simulink model "sbvf_model_2019b_local"  (R2019b)
settings: Solver=VariableStepAuto  StartTime=0.0  StopTime=Tsim  RelTol=1e-3
undefined symbols (not defined in the file): A0, Ad, B, C, c, D, F_local, Gdiag, k, K, L_leader, std_dev, x0, x0_leader
libraries: dspindex x54
settings Model: Creator=andre  LastModifiedBy=frare
settings DebuggingCC: UnconnectedInputMsg=none  UnconnectedOutputMsg=none  UnconnectedLineMsg=none
settings ModelReferenceCC: EnableRefExpFcnMdlSchedulingChecks=off
settings RTWCC: Description=Generic Real-Time Target

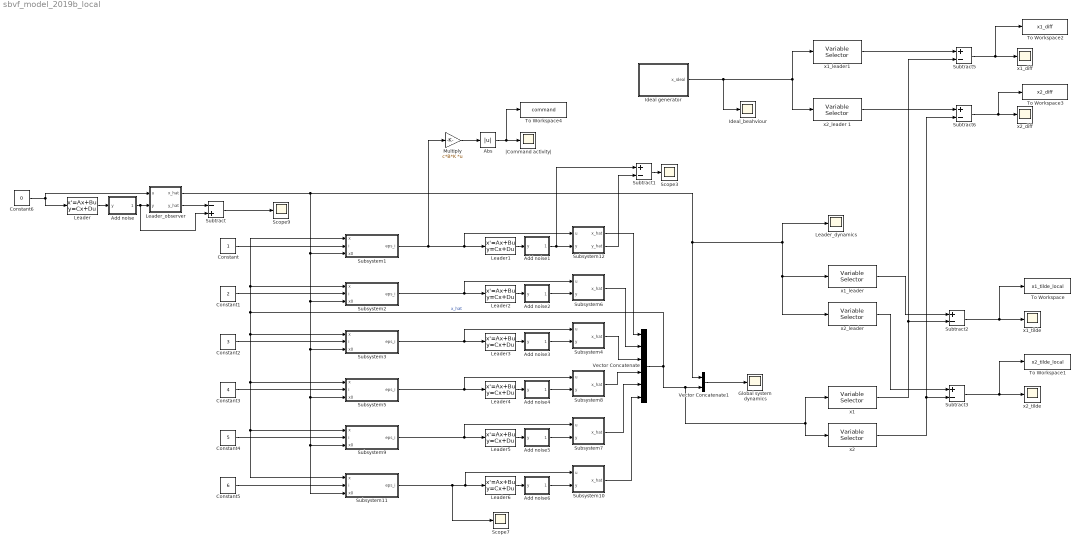
== system sbvf_model_2019b_local ==
  Abs : Abs
  Add noise : Subsystem
  Add noise1 : Subsystem
  Add noise2 : Subsystem
  Add noise3 : Subsystem
  Add noise4 : Subsystem
  Add noise5 : Subsystem
  Add noise6 : Subsystem
  Constant : Constant
  Constant1 : Constant  Value=2
  Constant2 : Constant  Value=3
  Constant3 : Constant  Value=4
  Constant4 : Constant  Value=5
  Constant5 : Constant  Value=6
  Constant6 : Constant  Value=0
  Global system dynamics : Scope
  "Ideal generator " : Subsystem
  "Ideal_beahviour " : Scope
  Leader : StateSpace  A=A0  B=B  C=C  D=0  InitialCondition=x0_leader
  Leader1 : StateSpace  A=A0  B=c*B*K  C=C  D=D  InitialCondition=x0(:,1)
  Leader2 : StateSpace  A=A0  B=c*B*K  C=C  D=D  InitialCondition=x0(:,2)
  Leader3 : StateSpace  A=A0  B=c*B*K  C=C  D=D  InitialCondition=x0(:,3)
  Leader4 : StateSpace  A=A0  B=c*B*K  C=C  D=D  InitialCondition=x0(:,4)
  Leader5 : StateSpace  A=A0  B=c*B*K  C=C  D=D  InitialCondition=x0(:,5)
  Leader6 : StateSpace  A=A0  B=c*B*K  C=C  D=D  InitialCondition=x0(:,6)
  "Leader_dynamics " : Scope
  Leader_observer : Subsystem
  Multiply : Gain  Gain=c*B*K  Multiplication=Matrix(K*u)
  Scope3 : Scope
  Scope7 : Scope
  Scope9 : Scope
  Subsystem1 : Subsystem
  Subsystem10 : Subsystem
  Subsystem11 : Subsystem
  Subsystem12 : Subsystem
  Subsystem2 : Subsystem
  Subsystem3 : Subsystem
  Subsystem4 : Subsystem
  Subsystem5 : Subsystem
  Subsystem6 : Subsystem
  Subsystem7 : Subsystem
  Subsystem8 : Subsystem
  Subsystem9 : Subsystem
  Subtract : Sum  Inputs=-+
  Subtract{1..3,5..6} (5 alike) : Sum  Inputs=+-
  To Workspace : ToWorkspace  VariableName=x1_tilde_local  SaveFormat=Timeseries  SampleTime=-1
  To Workspace1 : ToWorkspace  VariableName=x2_tilde_local  SaveFormat=Timeseries  SampleTime=-1
  To Workspace2 : ToWorkspace  VariableName=x1_diff  SaveFormat=Timeseries  SampleTime=-1
  To Workspace3 : ToWorkspace  VariableName=x2_diff  SaveFormat=Timeseries  SampleTime=-1
  To Workspace4 : ToWorkspace  VariableName=command  SaveFormat=Timeseries  SampleTime=-1
  Vector Concatenate : Concatenate  NumInputs=6  Mode=Multidimensional array  ConcatenateDimension=2
  Vector Concatenate1 : Concatenate  Mode=Multidimensional array  ConcatenateDimension=2
  "x1 " : dspindex/Variable Selector  NumInputs=1  rowsOrCols=Rows  IdxMode=Fixed  Elements=1  ZerOneIdxMode=One-based  errmode=Clip Index  FillMode=on  FillValues=0
  "x1_diff " : Scope
  x1_leader : dspindex/Variable Selector  NumInputs=1  rowsOrCols=Rows  IdxMode=Fixed  Elements=1  ZerOneIdxMode=One-based  errmode=Clip Index  FillMode=on  FillValues=0
  x1_leader1 : dspindex/Variable Selector  NumInputs=1  rowsOrCols=Rows  IdxMode=Fixed  Elements=1  ZerOneIdxMode=One-based  errmode=Clip Index  FillMode=on  FillValues=0
  x1_tilde : Scope
  x2 : dspindex/Variable Selector  NumInputs=1  rowsOrCols=Rows  IdxMode=Fixed  Elements=2  ZerOneIdxMode=One-based  errmode=Clip Index  FillMode=on  FillValues=0
  x2_diff : Scope
  "x2_leader " : dspindex/Variable Selector  NumInputs=1  rowsOrCols=Rows  IdxMode=Fixed  Elements=2  ZerOneIdxMode=One-based  errmode=Clip Index  FillMode=on  FillValues=0
  x2_leader 1 : dspindex/Variable Selector  NumInputs=1  rowsOrCols=Rows  IdxMode=Fixed  Elements=2  ZerOneIdxMode=One-based  errmode=Clip Index  FillMode=on  FillValues=0
  "x2_tilde " : Scope
  "|Command activity| " : Scope
  wires:
  Constant/1 -> Subsystem1/2(i)
  Constant1/1 -> Subsystem2/2(i)
  Constant3/1 -> Subsystem5/2(i)
  Constant5/1 -> Subsystem11/2(i)
  Constant4/1 -> Subsystem9/2(i)
  Constant2/1 -> Subsystem3/2(i)
  Leader/1 -> Add noise/1(y)
  Constant6/1 -> Leader/1, Leader_observer/1(u)
  Leader_observer/2(y_hat) -> Subtract/1
  Subsystem12/1(x_hat) -> Vector Concatenate/1
  Subsystem6/1(x_hat) -> Vector Concatenate/2
  Subsystem4/1(x_hat) -> Vector Concatenate/3
  Subsystem8/1(x_hat) -> Vector Concatenate/4
  Subsystem7/1(x_hat) -> Vector Concatenate/5
  Subsystem10/1(x_hat) -> Vector Concatenate/6
  Subsystem11/1(eps_i) -> Subsystem10/1(u), Leader6/1, Scope7/1
  Subtract/1 -> Scope9/1
  Leader1/1 -> Add noise1/1(y)
  Subsystem5/1(eps_i) -> Subsystem8/1(u), Leader4/1
  Subsystem9/1(eps_i) -> Subsystem7/1(u), Leader5/1
  Subsystem2/1(eps_i) -> Subsystem6/1(u), Leader2/1
  Subsystem3/1(eps_i) -> Subsystem4/1(u), Leader3/1
  Subsystem12/2("y_hat ") -> Subtract1/2
  Subtract1/1 -> Scope3/1
  Subtract2/1 -> To Workspace/1, x1_tilde/1
  Vector Concatenate/1 -> Subsystem11/1(x), Subsystem9/1(x), Subsystem5/1(x), Subsystem3/1(x), Subsystem1/1(x), Subsystem2/1(x), x2/1, "x1 "/1, Vector Concatenate1/2  "x_hat"
  Vector Concatenate1/1 -> Global system dynamics/1
  x1_leader/1 -> Subtract2/1
  Subtract3/1 -> To Workspace1/1, "x2_tilde "/1
  "x2_leader "/1 -> Subtract3/1
  Leader_observer/1(x_hat) -> Subsystem11/3(x0), Subsystem9/3(x0), Subsystem5/3(x0), Subsystem3/3(x0), Subsystem2/3(x0), Subsystem1/3(x0), "Leader_dynamics "/1, "x2_leader "/1, x1_leader/1, Vector Concatenate1/1
  Add noise1/1(y_noisy) -> Subtract1/1, Subsystem12/2("y ")
  Add noise2/1(y_noisy) -> Subsystem6/2("y ")
  Add noise3/1(y_noisy) -> Subsystem4/2("y ")
  Add noise4/1(y_noisy) -> Subsystem8/2("y ")
  Add noise5/1(y_noisy) -> Subsystem7/2("y ")
  Add noise6/1(y_noisy) -> Subsystem10/2("y ")
  Add noise/1(y_noisy) -> Subtract/2, Leader_observer/2("y ")
  Leader2/1 -> Add noise2/1(y)
  Leader4/1 -> Add noise4/1(y)
  Leader3/1 -> Add noise3/1(y)
  Leader6/1 -> Add noise6/1(y)
  Leader5/1 -> Add noise5/1(y)
  Subtract5/1 -> To Workspace2/1, "x1_diff "/1
  x2/1 -> Subtract6/2, Subtract3/2
  x1_leader1/1 -> Subtract5/1
  x2_leader 1/1 -> Subtract6/1
  "Ideal generator "/1("x_ideal ") -> "Ideal_beahviour "/1, x2_leader 1/1, x1_leader1/1
  "x1 "/1 -> Subtract5/2, Subtract2/2
  Subtract6/1 -> To Workspace3/1, x2_diff/1
  Abs/1 -> To Workspace4/1, "|Command activity| "/1
  Subsystem1/1(eps_i) -> Multiply/1, Subsystem12/1(u), Leader1/1
  Multiply/1 -> Abs/1

== system sbvf_model_2019b_local/Add noise ==
  y : Inport
  Random Number : RandomNumber  SampleTime=0.1
  Sum : Sum  Inputs=|++
  "std_dev(k) " : Gain  Gain=std_dev(k)
  y_noisy : Outport
  wires:
  Random Number/1 -> "std_dev(k) "/1
  y/1 -> Sum/1
  "std_dev(k) "/1 -> Sum/2
  Sum/1 -> y_noisy/1

== system sbvf_model_2019b_local/Add noise1 ==
  y : Inport
  Random Number : RandomNumber  SampleTime=0.1
  Sum : Sum  Inputs=|++
  "std_dev(k) " : Gain  Gain=std_dev(k)
  y_noisy : Outport
  wires:
  Random Number/1 -> "std_dev(k) "/1
  y/1 -> Sum/1
  "std_dev(k) "/1 -> Sum/2
  Sum/1 -> y_noisy/1

== system sbvf_model_2019b_local/Add noise2 ==
  y : Inport
  Random Number : RandomNumber  SampleTime=0.1
  Sum : Sum  Inputs=|++
  "std_dev(k) " : Gain  Gain=std_dev(k)
  y_noisy : Outport
  wires:
  Random Number/1 -> "std_dev(k) "/1
  y/1 -> Sum/1
  "std_dev(k) "/1 -> Sum/2
  Sum/1 -> y_noisy/1

== system sbvf_model_2019b_local/Add noise3 ==
  y : Inport
  Random Number : RandomNumber  SampleTime=0.1
  Sum : Sum  Inputs=|++
  "std_dev(k) " : Gain  Gain=std_dev(k)
  y_noisy : Outport
  wires:
  Random Number/1 -> "std_dev(k) "/1
  y/1 -> Sum/1
  "std_dev(k) "/1 -> Sum/2
  Sum/1 -> y_noisy/1

== system sbvf_model_2019b_local/Add noise4 ==
  y : Inport
  Random Number : RandomNumber  SampleTime=0.1
  Sum : Sum  Inputs=|++
  "std_dev(k) " : Gain  Gain=std_dev(k)
  y_noisy : Outport
  wires:
  Random Number/1 -> "std_dev(k) "/1
  y/1 -> Sum/1
  "std_dev(k) "/1 -> Sum/2
  Sum/1 -> y_noisy/1

== system sbvf_model_2019b_local/Add noise5 ==
  y : Inport
  Random Number : RandomNumber  SampleTime=0.1
  Sum : Sum  Inputs=|++
  "std_dev(k) " : Gain  Gain=std_dev(k)
  y_noisy : Outport
  wires:
  Random Number/1 -> "std_dev(k) "/1
  y/1 -> Sum/1
  "std_dev(k) "/1 -> Sum/2
  Sum/1 -> y_noisy/1

== system sbvf_model_2019b_local/Add noise6 ==
  y : Inport
  Random Number : RandomNumber  SampleTime=0.1
  Sum : Sum  Inputs=|++
  "std_dev(k) " : Gain  Gain=std_dev(k)
  y_noisy : Outport
  wires:
  Random Number/1 -> "std_dev(k) "/1
  y/1 -> Sum/1
  "std_dev(k) "/1 -> Sum/2
  Sum/1 -> y_noisy/1

== system sbvf_model_2019b_local/Ideal generator  ==
  Constant7 : Constant  Value=0
  Leader2 : StateSpace  A=A0  B=B  C=C  D=0  InitialCondition=x0_leader
  Subsystem14 : Subsystem
  "x_ideal " : Outport
  wires:
  Constant7/1 -> Subsystem14/1(u), Leader2/1
  Leader2/1 -> Subsystem14/2("y ")
  Subsystem14/1(x_hat) -> "x_ideal "/1

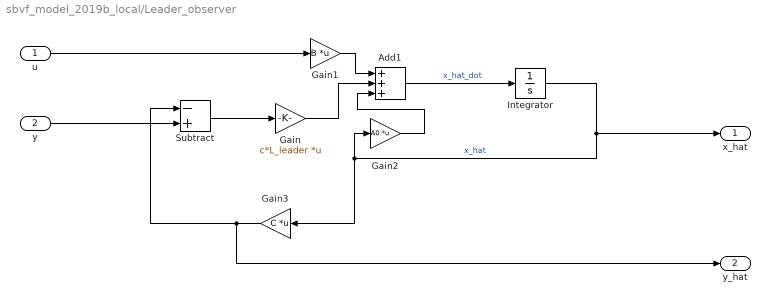
== system sbvf_model_2019b_local/Leader_observer ==
  u : Inport
  "y " : Inport  Port=2
  Add1 : Sum  Inputs=+++
  Gain : Gain  Gain=c*L_leader  Multiplication=Matrix(K*u)
  Gain1 : Gain  Gain=B  Multiplication=Matrix(K*u)
  Gain2 : Gain  Gain=A0  Multiplication=Matrix(K*u)
  Gain3 : Gain  Gain=C  Multiplication=Matrix(K*u)
  Integrator : Integrator  InitialCondition=x0_leader
  Subtract : Sum  Inputs=-+
  x_hat : Outport
  y_hat : Outport  Port=2
  wires:
  Gain2/1 -> Add1/3
  Gain/1 -> Add1/2
  Integrator/1 -> x_hat/1, Gain3/1, Gain2/1  "x_hat"
  Add1/1 -> Integrator/1  "x_hat_dot"
  u/1 -> Gain1/1
  Gain1/1 -> Add1/1
  "y "/1 -> Subtract/2
  Subtract/1 -> Gain/1
  Gain3/1 -> y_hat/1, Subtract/1

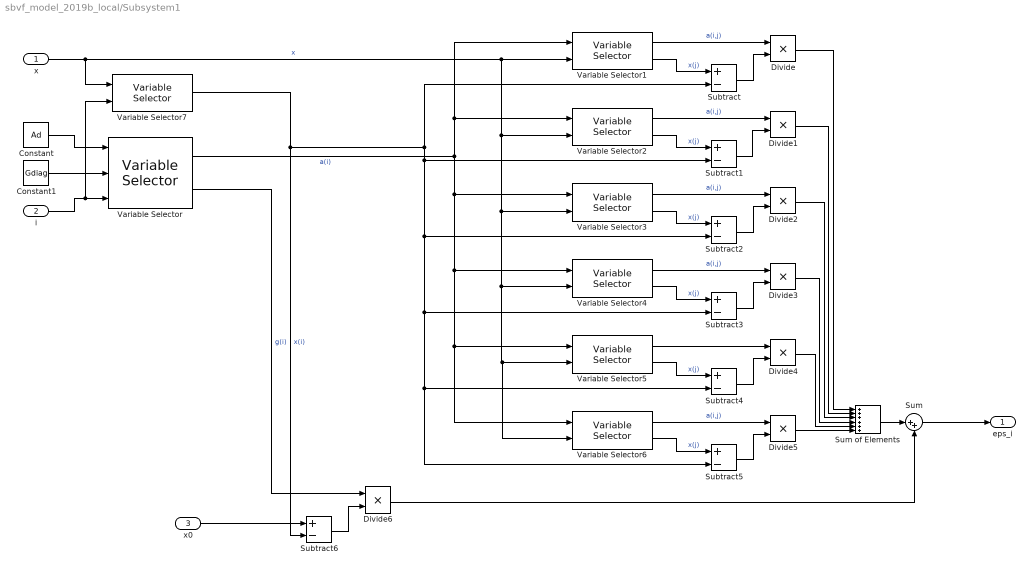
== system sbvf_model_2019b_local/Subsystem1 ==
  x : Inport
  i : Inport  Port=2
  x0 : Inport  Port=3
  Constant : Constant  Value=Ad
  Constant1 : Constant  Value=Gdiag
  Divide{,1..6} (7 alike) : Product
  Subtract{,1..6} (7 alike) : Sum  Inputs=+-
  Sum : Sum  Inputs=|++
  Sum of Elements : Sum  Inputs=++++++
  Variable Selector : dspindex/Variable Selector  NumInputs=2  rowsOrCols=Rows  IdxMode=Variable  Elements=[1 3]  ZerOneIdxMode=One-based  errmode=Clip and Warn  FillMode=on  FillValues=0
  Variable Selector1 : dspindex/Variable Selector  NumInputs=2  rowsOrCols=Columns  IdxMode=Fixed  Elements=1  ZerOneIdxMode=One-based  errmode=Generate Error  FillMode=on  FillValues=0
  Variable Selector2 : dspindex/Variable Selector  NumInputs=2  rowsOrCols=Columns  IdxMode=Fixed  Elements=2  ZerOneIdxMode=One-based  errmode=Generate Error  FillMode=on  FillValues=0
  Variable Selector3 : dspindex/Variable Selector  NumInputs=2  rowsOrCols=Columns  IdxMode=Fixed  Elements=3  ZerOneIdxMode=One-based  errmode=Generate Error  FillMode=on  FillValues=0
  Variable Selector4 : dspindex/Variable Selector  NumInputs=2  rowsOrCols=Columns  IdxMode=Fixed  Elements=4  ZerOneIdxMode=One-based  errmode=Generate Error  FillMode=on  FillValues=0
  Variable Selector5 : dspindex/Variable Selector  NumInputs=2  rowsOrCols=Columns  IdxMode=Fixed  Elements=5  ZerOneIdxMode=One-based  errmode=Generate Error  FillMode=on  FillValues=0
  Variable Selector6 : dspindex/Variable Selector  NumInputs=2  rowsOrCols=Columns  IdxMode=Fixed  Elements=6  ZerOneIdxMode=One-based  errmode=Generate Error  FillMode=on  FillValues=0
  Variable Selector7 : dspindex/Variable Selector  NumInputs=1  rowsOrCols=Columns  IdxMode=Variable  Elements=1  ZerOneIdxMode=One-based  errmode=Generate Error  FillMode=on  FillValues=0
  eps_i : Outport
  wires:
  Variable Selector/1 -> Variable Selector3/1, Variable Selector4/1, Variable Selector6/1, Variable Selector5/1, Variable Selector2/1, Variable Selector1/1  "a(i)"
  x/1 -> Variable Selector7/1, Variable Selector2/2, Variable Selector3/2, Variable Selector4/2, Variable Selector6/2, Variable Selector5/2, Variable Selector1/2  "x"
  Constant/1 -> Variable Selector/1
  i/1 -> Variable Selector7/2, Variable Selector/3
  Variable Selector1/1 -> Divide/1  "a(i,j)"
  Variable Selector1/2 -> Subtract/1  "x(j)"
  Subtract/1 -> Divide/2
  Variable Selector2/2 -> Subtract1/1  "x(j)"
  Variable Selector2/1 -> Divide1/1  "a(i,j)"
  Subtract1/1 -> Divide1/2
  Variable Selector3/1 -> Divide2/1  "a(i,j)"
  Variable Selector3/2 -> Subtract2/1  "x(j)"
  Subtract2/1 -> Divide2/2
  Variable Selector4/1 -> Divide3/1  "a(i,j)"
  Variable Selector4/2 -> Subtract3/1  "x(j)"
  Subtract3/1 -> Divide3/2
  Variable Selector5/2 -> Subtract4/1  "x(j)"
  Subtract4/1 -> Divide4/2
  Variable Selector5/1 -> Divide4/1
  Variable Selector6/1 -> Divide5/1  "a(i,j)"
  Variable Selector7/1 -> Subtract6/2, Subtract5/2, Subtract4/2, Subtract3/2, Subtract2/2, Subtract1/2, Subtract/2  "x(i)"
  Variable Selector6/2 -> Subtract5/1  "x(j)"
  Subtract5/1 -> Divide5/2
  Divide2/1 -> Sum of Elements/3
  Divide1/1 -> Sum of Elements/2
  Divide5/1 -> Sum of Elements/6
  Divide4/1 -> Sum of Elements/5
  Divide3/1 -> Sum of Elements/4
  Divide/1 -> Sum of Elements/1
  Variable Selector/2 -> Divide6/1  "g(i)"
  Subtract6/1 -> Divide6/2
  x0/1 -> Subtract6/1
  Divide6/1 -> Sum/2
  Sum of Elements/1 -> Sum/1
  Sum/1 -> eps_i/1
  Constant1/1 -> Variable Selector/2

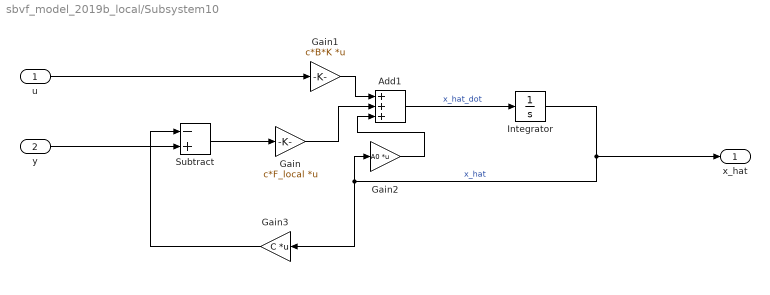
== system sbvf_model_2019b_local/Subsystem10 ==
  u : Inport
  "y " : Inport  Port=2
  Add1 : Sum  Inputs=+++
  Gain : Gain  Gain=c*F_local  Multiplication=Matrix(K*u)
  Gain1 : Gain  Gain=c*B*K  Multiplication=Matrix(K*u)
  Gain2 : Gain  Gain=A0  Multiplication=Matrix(K*u)
  Gain3 : Gain  Gain=C  Multiplication=Matrix(K*u)
  Integrator : Integrator  InitialCondition=x0(:,6)
  Subtract : Sum  Inputs=-+
  x_hat : Outport
  wires:
  Gain2/1 -> Add1/3
  Gain/1 -> Add1/2
  Integrator/1 -> x_hat/1, Gain3/1, Gain2/1  "x_hat"
  Add1/1 -> Integrator/1  "x_hat_dot"
  u/1 -> Gain1/1
  Gain1/1 -> Add1/1
  "y "/1 -> Subtract/2
  Subtract/1 -> Gain/1
  Gain3/1 -> Subtract/1

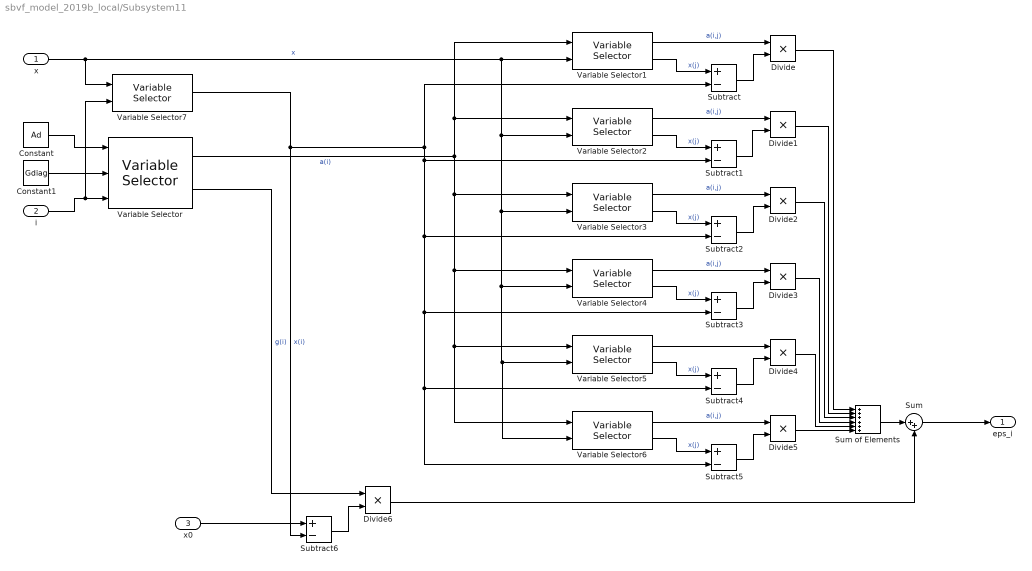
== system sbvf_model_2019b_local/Subsystem11 ==
  x : Inport
  i : Inport  Port=2
  x0 : Inport  Port=3
  Constant : Constant  Value=Ad
  Constant1 : Constant  Value=Gdiag
  Divide{,1..6} (7 alike) : Product
  Subtract{,1..6} (7 alike) : Sum  Inputs=+-
  Sum : Sum  Inputs=|++
  Sum of Elements : Sum  Inputs=++++++
  Variable Selector : dspindex/Variable Selector  NumInputs=2  rowsOrCols=Rows  IdxMode=Variable  Elements=[1 3]  ZerOneIdxMode=One-based  errmode=Clip and Warn  FillMode=on  FillValues=0
  Variable Selector1 : dspindex/Variable Selector  NumInputs=2  rowsOrCols=Columns  IdxMode=Fixed  Elements=1  ZerOneIdxMode=One-based  errmode=Generate Error  FillMode=on  FillValues=0
  Variable Selector2 : dspindex/Variable Selector  NumInputs=2  rowsOrCols=Columns  IdxMode=Fixed  Elements=2  ZerOneIdxMode=One-based  errmode=Generate Error  FillMode=on  FillValues=0
  Variable Selector3 : dspindex/Variable Selector  NumInputs=2  rowsOrCols=Columns  IdxMode=Fixed  Elements=3  ZerOneIdxMode=One-based  errmode=Generate Error  FillMode=on  FillValues=0
  Variable Selector4 : dspindex/Variable Selector  NumInputs=2  rowsOrCols=Columns  IdxMode=Fixed  Elements=4  ZerOneIdxMode=One-based  errmode=Generate Error  FillMode=on  FillValues=0
  Variable Selector5 : dspindex/Variable Selector  NumInputs=2  rowsOrCols=Columns  IdxMode=Fixed  Elements=5  ZerOneIdxMode=One-based  errmode=Generate Error  FillMode=on  FillValues=0
  Variable Selector6 : dspindex/Variable Selector  NumInputs=2  rowsOrCols=Columns  IdxMode=Fixed  Elements=6  ZerOneIdxMode=One-based  errmode=Generate Error  FillMode=on  FillValues=0
  Variable Selector7 : dspindex/Variable Selector  NumInputs=1  rowsOrCols=Columns  IdxMode=Variable  Elements=1  ZerOneIdxMode=One-based  errmode=Generate Error  FillMode=on  FillValues=0
  eps_i : Outport
  wires:
  Variable Selector/1 -> Variable Selector3/1, Variable Selector4/1, Variable Selector6/1, Variable Selector5/1, Variable Selector2/1, Variable Selector1/1  "a(i)"
  x/1 -> Variable Selector7/1, Variable Selector2/2, Variable Selector3/2, Variable Selector4/2, Variable Selector6/2, Variable Selector5/2, Variable Selector1/2  "x"
  Constant/1 -> Variable Selector/1
  i/1 -> Variable Selector7/2, Variable Selector/3
  Variable Selector1/1 -> Divide/1  "a(i,j)"
  Variable Selector1/2 -> Subtract/1  "x(j)"
  Subtract/1 -> Divide/2
  Variable Selector2/2 -> Subtract1/1  "x(j)"
  Variable Selector2/1 -> Divide1/1  "a(i,j)"
  Subtract1/1 -> Divide1/2
  Variable Selector3/1 -> Divide2/1  "a(i,j)"
  Variable Selector3/2 -> Subtract2/1  "x(j)"
  Subtract2/1 -> Divide2/2
  Variable Selector4/1 -> Divide3/1  "a(i,j)"
  Variable Selector4/2 -> Subtract3/1  "x(j)"
  Subtract3/1 -> Divide3/2
  Variable Selector5/2 -> Subtract4/1  "x(j)"
  Subtract4/1 -> Divide4/2
  Variable Selector5/1 -> Divide4/1
  Variable Selector6/1 -> Divide5/1  "a(i,j)"
  Variable Selector7/1 -> Subtract6/2, Subtract5/2, Subtract4/2, Subtract3/2, Subtract2/2, Subtract1/2, Subtract/2  "x(i)"
  Variable Selector6/2 -> Subtract5/1  "x(j)"
  Subtract5/1 -> Divide5/2
  Divide2/1 -> Sum of Elements/3
  Divide1/1 -> Sum of Elements/2
  Divide5/1 -> Sum of Elements/6
  Divide4/1 -> Sum of Elements/5
  Divide3/1 -> Sum of Elements/4
  Divide/1 -> Sum of Elements/1
  Variable Selector/2 -> Divide6/1  "g(i)"
  Subtract6/1 -> Divide6/2
  x0/1 -> Subtract6/1
  Divide6/1 -> Sum/2
  Sum of Elements/1 -> Sum/1
  Sum/1 -> eps_i/1
  Constant1/1 -> Variable Selector/2

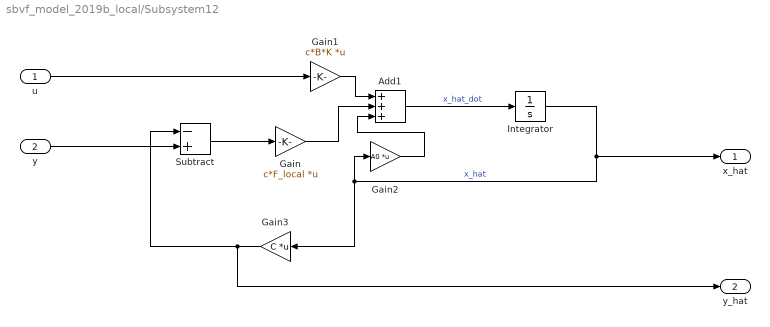
== system sbvf_model_2019b_local/Subsystem12 ==
  u : Inport
  "y " : Inport  Port=2
  Add1 : Sum  Inputs=+++
  Gain : Gain  Gain=c*F_local  Multiplication=Matrix(K*u)
  Gain1 : Gain  Gain=c*B*K  Multiplication=Matrix(K*u)
  Gain2 : Gain  Gain=A0  Multiplication=Matrix(K*u)
  Gain3 : Gain  Gain=C  Multiplication=Matrix(K*u)
  Integrator : Integrator  InitialCondition=x0(:,1)
  Subtract : Sum  Inputs=-+
  x_hat : Outport
  "y_hat " : Outport  Port=2
  wires:
  Gain2/1 -> Add1/3
  Gain/1 -> Add1/2
  Integrator/1 -> x_hat/1, Gain3/1, Gain2/1  "x_hat"
  Add1/1 -> Integrator/1  "x_hat_dot"
  u/1 -> Gain1/1
  Gain1/1 -> Add1/1
  "y "/1 -> Subtract/2
  Subtract/1 -> Gain/1
  Gain3/1 -> "y_hat "/1, Subtract/1

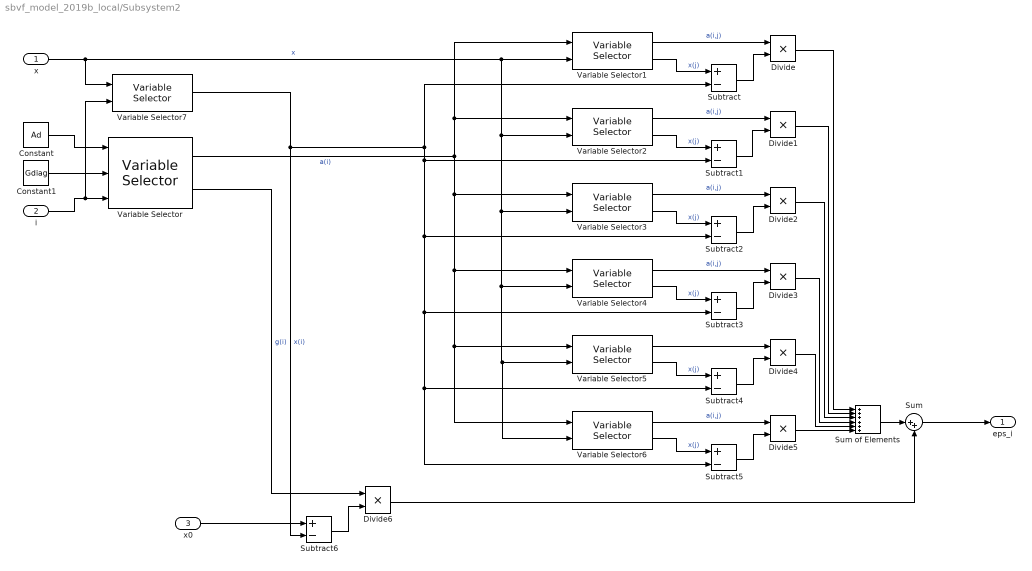
== system sbvf_model_2019b_local/Subsystem2 ==
  x : Inport
  i : Inport  Port=2
  x0 : Inport  Port=3
  Constant : Constant  Value=Ad
  Constant1 : Constant  Value=Gdiag
  Divide{,1..6} (7 alike) : Product
  Subtract{,1..6} (7 alike) : Sum  Inputs=+-
  Sum : Sum  Inputs=|++
  Sum of Elements : Sum  Inputs=++++++
  Variable Selector : dspindex/Variable Selector  NumInputs=2  rowsOrCols=Rows  IdxMode=Variable  Elements=[1 3]  ZerOneIdxMode=One-based  errmode=Clip and Warn  FillMode=on  FillValues=0
  Variable Selector1 : dspindex/Variable Selector  NumInputs=2  rowsOrCols=Columns  IdxMode=Fixed  Elements=1  ZerOneIdxMode=One-based  errmode=Generate Error  FillMode=on  FillValues=0
  Variable Selector2 : dspindex/Variable Selector  NumInputs=2  rowsOrCols=Columns  IdxMode=Fixed  Elements=2  ZerOneIdxMode=One-based  errmode=Generate Error  FillMode=on  FillValues=0
  Variable Selector3 : dspindex/Variable Selector  NumInputs=2  rowsOrCols=Columns  IdxMode=Fixed  Elements=3  ZerOneIdxMode=One-based  errmode=Generate Error  FillMode=on  FillValues=0
  Variable Selector4 : dspindex/Variable Selector  NumInputs=2  rowsOrCols=Columns  IdxMode=Fixed  Elements=4  ZerOneIdxMode=One-based  errmode=Generate Error  FillMode=on  FillValues=0
  Variable Selector5 : dspindex/Variable Selector  NumInputs=2  rowsOrCols=Columns  IdxMode=Fixed  Elements=5  ZerOneIdxMode=One-based  errmode=Generate Error  FillMode=on  FillValues=0
  Variable Selector6 : dspindex/Variable Selector  NumInputs=2  rowsOrCols=Columns  IdxMode=Fixed  Elements=6  ZerOneIdxMode=One-based  errmode=Generate Error  FillMode=on  FillValues=0
  Variable Selector7 : dspindex/Variable Selector  NumInputs=1  rowsOrCols=Columns  IdxMode=Variable  Elements=1  ZerOneIdxMode=One-based  errmode=Generate Error  FillMode=on  FillValues=0
  eps_i : Outport
  wires:
  Variable Selector/1 -> Variable Selector3/1, Variable Selector4/1, Variable Selector6/1, Variable Selector5/1, Variable Selector2/1, Variable Selector1/1  "a(i)"
  x/1 -> Variable Selector7/1, Variable Selector2/2, Variable Selector3/2, Variable Selector4/2, Variable Selector6/2, Variable Selector5/2, Variable Selector1/2  "x"
  Constant/1 -> Variable Selector/1
  i/1 -> Variable Selector7/2, Variable Selector/3
  Variable Selector1/1 -> Divide/1  "a(i,j)"
  Variable Selector1/2 -> Subtract/1  "x(j)"
  Subtract/1 -> Divide/2
  Variable Selector2/2 -> Subtract1/1  "x(j)"
  Variable Selector2/1 -> Divide1/1  "a(i,j)"
  Subtract1/1 -> Divide1/2
  Variable Selector3/1 -> Divide2/1  "a(i,j)"
  Variable Selector3/2 -> Subtract2/1  "x(j)"
  Subtract2/1 -> Divide2/2
  Variable Selector4/1 -> Divide3/1  "a(i,j)"
  Variable Selector4/2 -> Subtract3/1  "x(j)"
  Subtract3/1 -> Divide3/2
  Variable Selector5/2 -> Subtract4/1  "x(j)"
  Subtract4/1 -> Divide4/2
  Variable Selector5/1 -> Divide4/1
  Variable Selector6/1 -> Divide5/1  "a(i,j)"
  Variable Selector7/1 -> Subtract6/2, Subtract5/2, Subtract4/2, Subtract3/2, Subtract2/2, Subtract1/2, Subtract/2  "x(i)"
  Variable Selector6/2 -> Subtract5/1  "x(j)"
  Subtract5/1 -> Divide5/2
  Divide2/1 -> Sum of Elements/3
  Divide1/1 -> Sum of Elements/2
  Divide5/1 -> Sum of Elements/6
  Divide4/1 -> Sum of Elements/5
  Divide3/1 -> Sum of Elements/4
  Divide/1 -> Sum of Elements/1
  Variable Selector/2 -> Divide6/1  "g(i)"
  Subtract6/1 -> Divide6/2
  x0/1 -> Subtract6/1
  Divide6/1 -> Sum/2
  Sum of Elements/1 -> Sum/1
  Sum/1 -> eps_i/1
  Constant1/1 -> Variable Selector/2

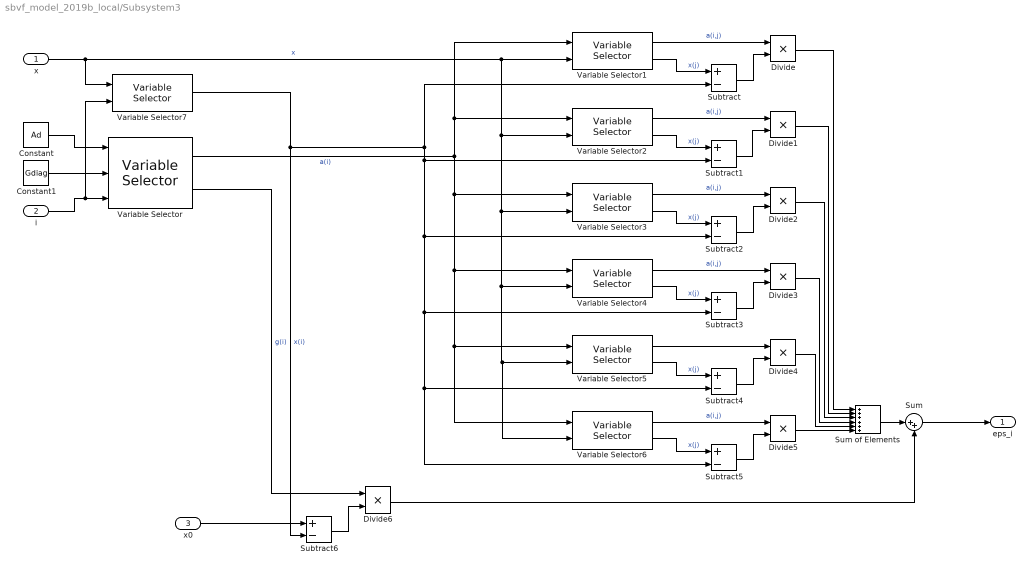
== system sbvf_model_2019b_local/Subsystem3 ==
  x : Inport
  i : Inport  Port=2
  x0 : Inport  Port=3
  Constant : Constant  Value=Ad
  Constant1 : Constant  Value=Gdiag
  Divide{,1..6} (7 alike) : Product
  Subtract{,1..6} (7 alike) : Sum  Inputs=+-
  Sum : Sum  Inputs=|++
  Sum of Elements : Sum  Inputs=++++++
  Variable Selector : dspindex/Variable Selector  NumInputs=2  rowsOrCols=Rows  IdxMode=Variable  Elements=[1 3]  ZerOneIdxMode=One-based  errmode=Clip and Warn  FillMode=on  FillValues=0
  Variable Selector1 : dspindex/Variable Selector  NumInputs=2  rowsOrCols=Columns  IdxMode=Fixed  Elements=1  ZerOneIdxMode=One-based  errmode=Generate Error  FillMode=on  FillValues=0
  Variable Selector2 : dspindex/Variable Selector  NumInputs=2  rowsOrCols=Columns  IdxMode=Fixed  Elements=2  ZerOneIdxMode=One-based  errmode=Generate Error  FillMode=on  FillValues=0
  Variable Selector3 : dspindex/Variable Selector  NumInputs=2  rowsOrCols=Columns  IdxMode=Fixed  Elements=3  ZerOneIdxMode=One-based  errmode=Generate Error  FillMode=on  FillValues=0
  Variable Selector4 : dspindex/Variable Selector  NumInputs=2  rowsOrCols=Columns  IdxMode=Fixed  Elements=4  ZerOneIdxMode=One-based  errmode=Generate Error  FillMode=on  FillValues=0
  Variable Selector5 : dspindex/Variable Selector  NumInputs=2  rowsOrCols=Columns  IdxMode=Fixed  Elements=5  ZerOneIdxMode=One-based  errmode=Generate Error  FillMode=on  FillValues=0
  Variable Selector6 : dspindex/Variable Selector  NumInputs=2  rowsOrCols=Columns  IdxMode=Fixed  Elements=6  ZerOneIdxMode=One-based  errmode=Generate Error  FillMode=on  FillValues=0
  Variable Selector7 : dspindex/Variable Selector  NumInputs=1  rowsOrCols=Columns  IdxMode=Variable  Elements=1  ZerOneIdxMode=One-based  errmode=Generate Error  FillMode=on  FillValues=0
  eps_i : Outport
  wires:
  Variable Selector/1 -> Variable Selector3/1, Variable Selector4/1, Variable Selector6/1, Variable Selector5/1, Variable Selector2/1, Variable Selector1/1  "a(i)"
  x/1 -> Variable Selector7/1, Variable Selector2/2, Variable Selector3/2, Variable Selector4/2, Variable Selector6/2, Variable Selector5/2, Variable Selector1/2  "x"
  Constant/1 -> Variable Selector/1
  i/1 -> Variable Selector7/2, Variable Selector/3
  Variable Selector1/1 -> Divide/1  "a(i,j)"
  Variable Selector1/2 -> Subtract/1  "x(j)"
  Subtract/1 -> Divide/2
  Variable Selector2/2 -> Subtract1/1  "x(j)"
  Variable Selector2/1 -> Divide1/1  "a(i,j)"
  Subtract1/1 -> Divide1/2
  Variable Selector3/1 -> Divide2/1  "a(i,j)"
  Variable Selector3/2 -> Subtract2/1  "x(j)"
  Subtract2/1 -> Divide2/2
  Variable Selector4/1 -> Divide3/1  "a(i,j)"
  Variable Selector4/2 -> Subtract3/1  "x(j)"
  Subtract3/1 -> Divide3/2
  Variable Selector5/2 -> Subtract4/1  "x(j)"
  Subtract4/1 -> Divide4/2
  Variable Selector5/1 -> Divide4/1
  Variable Selector6/1 -> Divide5/1  "a(i,j)"
  Variable Selector7/1 -> Subtract6/2, Subtract5/2, Subtract4/2, Subtract3/2, Subtract2/2, Subtract1/2, Subtract/2  "x(i)"
  Variable Selector6/2 -> Subtract5/1  "x(j)"
  Subtract5/1 -> Divide5/2
  Divide2/1 -> Sum of Elements/3
  Divide1/1 -> Sum of Elements/2
  Divide5/1 -> Sum of Elements/6
  Divide4/1 -> Sum of Elements/5
  Divide3/1 -> Sum of Elements/4
  Divide/1 -> Sum of Elements/1
  Variable Selector/2 -> Divide6/1  "g(i)"
  Subtract6/1 -> Divide6/2
  x0/1 -> Subtract6/1
  Divide6/1 -> Sum/2
  Sum of Elements/1 -> Sum/1
  Sum/1 -> eps_i/1
  Constant1/1 -> Variable Selector/2

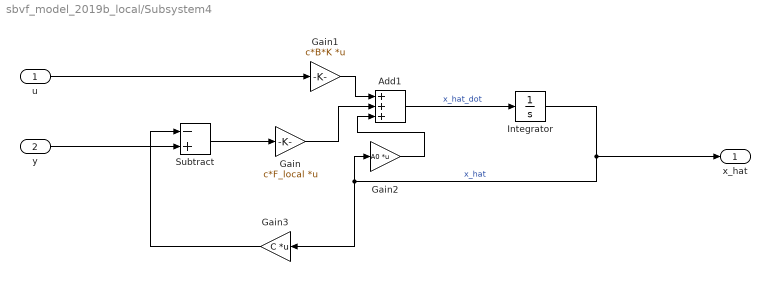
== system sbvf_model_2019b_local/Subsystem4 ==
  u : Inport
  "y " : Inport  Port=2
  Add1 : Sum  Inputs=+++
  Gain : Gain  Gain=c*F_local  Multiplication=Matrix(K*u)
  Gain1 : Gain  Gain=c*B*K  Multiplication=Matrix(K*u)
  Gain2 : Gain  Gain=A0  Multiplication=Matrix(K*u)
  Gain3 : Gain  Gain=C  Multiplication=Matrix(K*u)
  Integrator : Integrator  InitialCondition=x0(:,3)
  Subtract : Sum  Inputs=-+
  x_hat : Outport
  wires:
  Gain2/1 -> Add1/3
  Gain/1 -> Add1/2
  Integrator/1 -> x_hat/1, Gain3/1, Gain2/1  "x_hat"
  Add1/1 -> Integrator/1  "x_hat_dot"
  u/1 -> Gain1/1
  Gain1/1 -> Add1/1
  "y "/1 -> Subtract/2
  Subtract/1 -> Gain/1
  Gain3/1 -> Subtract/1

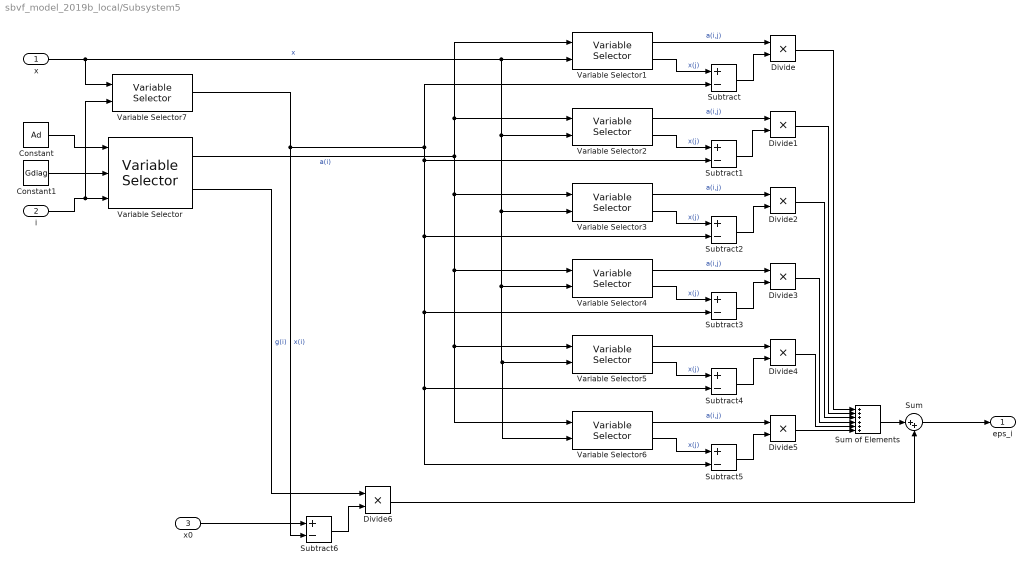
== system sbvf_model_2019b_local/Subsystem5 ==
  x : Inport
  i : Inport  Port=2
  x0 : Inport  Port=3
  Constant : Constant  Value=Ad
  Constant1 : Constant  Value=Gdiag
  Divide{,1..6} (7 alike) : Product
  Subtract{,1..6} (7 alike) : Sum  Inputs=+-
  Sum : Sum  Inputs=|++
  Sum of Elements : Sum  Inputs=++++++
  Variable Selector : dspindex/Variable Selector  NumInputs=2  rowsOrCols=Rows  IdxMode=Variable  Elements=[1 3]  ZerOneIdxMode=One-based  errmode=Clip and Warn  FillMode=on  FillValues=0
  Variable Selector1 : dspindex/Variable Selector  NumInputs=2  rowsOrCols=Columns  IdxMode=Fixed  Elements=1  ZerOneIdxMode=One-based  errmode=Generate Error  FillMode=on  FillValues=0
  Variable Selector2 : dspindex/Variable Selector  NumInputs=2  rowsOrCols=Columns  IdxMode=Fixed  Elements=2  ZerOneIdxMode=One-based  errmode=Generate Error  FillMode=on  FillValues=0
  Variable Selector3 : dspindex/Variable Selector  NumInputs=2  rowsOrCols=Columns  IdxMode=Fixed  Elements=3  ZerOneIdxMode=One-based  errmode=Generate Error  FillMode=on  FillValues=0
  Variable Selector4 : dspindex/Variable Selector  NumInputs=2  rowsOrCols=Columns  IdxMode=Fixed  Elements=4  ZerOneIdxMode=One-based  errmode=Generate Error  FillMode=on  FillValues=0
  Variable Selector5 : dspindex/Variable Selector  NumInputs=2  rowsOrCols=Columns  IdxMode=Fixed  Elements=5  ZerOneIdxMode=One-based  errmode=Generate Error  FillMode=on  FillValues=0
  Variable Selector6 : dspindex/Variable Selector  NumInputs=2  rowsOrCols=Columns  IdxMode=Fixed  Elements=6  ZerOneIdxMode=One-based  errmode=Generate Error  FillMode=on  FillValues=0
  Variable Selector7 : dspindex/Variable Selector  NumInputs=1  rowsOrCols=Columns  IdxMode=Variable  Elements=1  ZerOneIdxMode=One-based  errmode=Generate Error  FillMode=on  FillValues=0
  eps_i : Outport
  wires:
  Variable Selector/1 -> Variable Selector3/1, Variable Selector4/1, Variable Selector6/1, Variable Selector5/1, Variable Selector2/1, Variable Selector1/1  "a(i)"
  x/1 -> Variable Selector7/1, Variable Selector2/2, Variable Selector3/2, Variable Selector4/2, Variable Selector6/2, Variable Selector5/2, Variable Selector1/2  "x"
  Constant/1 -> Variable Selector/1
  i/1 -> Variable Selector7/2, Variable Selector/3
  Variable Selector1/1 -> Divide/1  "a(i,j)"
  Variable Selector1/2 -> Subtract/1  "x(j)"
  Subtract/1 -> Divide/2
  Variable Selector2/2 -> Subtract1/1  "x(j)"
  Variable Selector2/1 -> Divide1/1  "a(i,j)"
  Subtract1/1 -> Divide1/2
  Variable Selector3/1 -> Divide2/1  "a(i,j)"
  Variable Selector3/2 -> Subtract2/1  "x(j)"
  Subtract2/1 -> Divide2/2
  Variable Selector4/1 -> Divide3/1  "a(i,j)"
  Variable Selector4/2 -> Subtract3/1  "x(j)"
  Subtract3/1 -> Divide3/2
  Variable Selector5/2 -> Subtract4/1  "x(j)"
  Subtract4/1 -> Divide4/2
  Variable Selector5/1 -> Divide4/1
  Variable Selector6/1 -> Divide5/1  "a(i,j)"
  Variable Selector7/1 -> Subtract6/2, Subtract5/2, Subtract4/2, Subtract3/2, Subtract2/2, Subtract1/2, Subtract/2  "x(i)"
  Variable Selector6/2 -> Subtract5/1  "x(j)"
  Subtract5/1 -> Divide5/2
  Divide2/1 -> Sum of Elements/3
  Divide1/1 -> Sum of Elements/2
  Divide5/1 -> Sum of Elements/6
  Divide4/1 -> Sum of Elements/5
  Divide3/1 -> Sum of Elements/4
  Divide/1 -> Sum of Elements/1
  Variable Selector/2 -> Divide6/1  "g(i)"
  Subtract6/1 -> Divide6/2
  x0/1 -> Subtract6/1
  Divide6/1 -> Sum/2
  Sum of Elements/1 -> Sum/1
  Sum/1 -> eps_i/1
  Constant1/1 -> Variable Selector/2

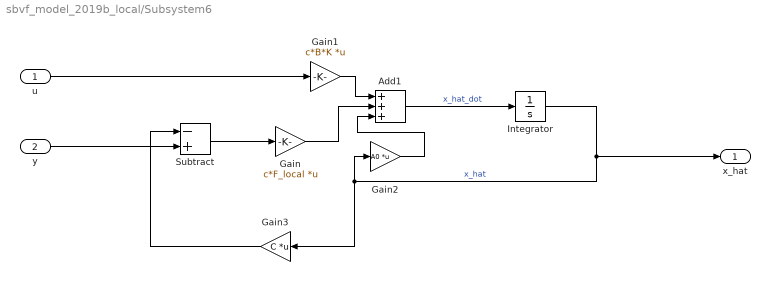
== system sbvf_model_2019b_local/Subsystem6 ==
  u : Inport
  "y " : Inport  Port=2
  Add1 : Sum  Inputs=+++
  Gain : Gain  Gain=c*F_local  Multiplication=Matrix(K*u)
  Gain1 : Gain  Gain=c*B*K  Multiplication=Matrix(K*u)
  Gain2 : Gain  Gain=A0  Multiplication=Matrix(K*u)
  Gain3 : Gain  Gain=C  Multiplication=Matrix(K*u)
  Integrator : Integrator  InitialCondition=x0(:,2)
  Subtract : Sum  Inputs=-+
  x_hat : Outport
  wires:
  Gain3/1 -> Subtract/1
  Subtract/1 -> Gain/1
  "y "/1 -> Subtract/2
  Gain1/1 -> Add1/1
  u/1 -> Gain1/1
  Add1/1 -> Integrator/1  "x_hat_dot"
  Integrator/1 -> Gain2/1, Gain3/1, x_hat/1  "x_hat"
  Gain/1 -> Add1/2
  Gain2/1 -> Add1/3

== system sbvf_model_2019b_local/Subsystem7 ==
  u : Inport
  "y " : Inport  Port=2
  Add1 : Sum  Inputs=+++
  Gain : Gain  Gain=c*F_local  Multiplication=Matrix(K*u)
  Gain1 : Gain  Gain=c*B*K  Multiplication=Matrix(K*u)
  Gain2 : Gain  Gain=A0  Multiplication=Matrix(K*u)
  Gain3 : Gain  Gain=C  Multiplication=Matrix(K*u)
  Integrator : Integrator  InitialCondition=x0(:,5)
  Subtract : Sum  Inputs=-+
  x_hat : Outport
  wires:
  Gain2/1 -> Add1/3
  Gain/1 -> Add1/2
  Integrator/1 -> x_hat/1, Gain3/1, Gain2/1  "x_hat"
  Add1/1 -> Integrator/1  "x_hat_dot"
  u/1 -> Gain1/1
  Gain1/1 -> Add1/1
  "y "/1 -> Subtract/2
  Subtract/1 -> Gain/1
  Gain3/1 -> Subtract/1

== system sbvf_model_2019b_local/Subsystem8 ==
  u : Inport
  "y " : Inport  Port=2
  Add1 : Sum  Inputs=+++
  Gain : Gain  Gain=c*F_local  Multiplication=Matrix(K*u)
  Gain1 : Gain  Gain=c*B*K  Multiplication=Matrix(K*u)
  Gain2 : Gain  Gain=A0  Multiplication=Matrix(K*u)
  Gain3 : Gain  Gain=C  Multiplication=Matrix(K*u)
  Integrator : Integrator  InitialCondition=x0(:,4)
  Subtract : Sum  Inputs=-+
  x_hat : Outport
  wires:
  Gain3/1 -> Subtract/1
  Subtract/1 -> Gain/1
  "y "/1 -> Subtract/2
  Gain1/1 -> Add1/1
  u/1 -> Gain1/1
  Add1/1 -> Integrator/1  "x_hat_dot"
  Integrator/1 -> Gain2/1, Gain3/1, x_hat/1  "x_hat"
  Gain/1 -> Add1/2
  Gain2/1 -> Add1/3

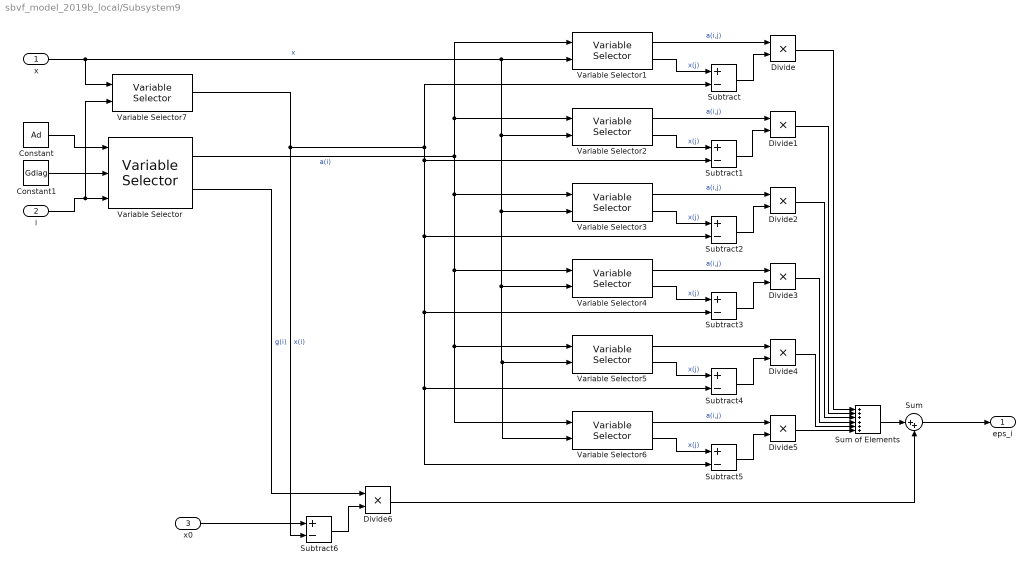
== system sbvf_model_2019b_local/Subsystem9 ==
  x : Inport
  i : Inport  Port=2
  x0 : Inport  Port=3
  Constant : Constant  Value=Ad
  Constant1 : Constant  Value=Gdiag
  Divide{,1..6} (7 alike) : Product
  Subtract{,1..6} (7 alike) : Sum  Inputs=+-
  Sum : Sum  Inputs=|++
  Sum of Elements : Sum  Inputs=++++++
  Variable Selector : dspindex/Variable Selector  NumInputs=2  rowsOrCols=Rows  IdxMode=Variable  Elements=[1 3]  ZerOneIdxMode=One-based  errmode=Clip and Warn  FillMode=on  FillValues=0
  Variable Selector1 : dspindex/Variable Selector  NumInputs=2  rowsOrCols=Columns  IdxMode=Fixed  Elements=1  ZerOneIdxMode=One-based  errmode=Generate Error  FillMode=on  FillValues=0
  Variable Selector2 : dspindex/Variable Selector  NumInputs=2  rowsOrCols=Columns  IdxMode=Fixed  Elements=2  ZerOneIdxMode=One-based  errmode=Generate Error  FillMode=on  FillValues=0
  Variable Selector3 : dspindex/Variable Selector  NumInputs=2  rowsOrCols=Columns  IdxMode=Fixed  Elements=3  ZerOneIdxMode=One-based  errmode=Generate Error  FillMode=on  FillValues=0
  Variable Selector4 : dspindex/Variable Selector  NumInputs=2  rowsOrCols=Columns  IdxMode=Fixed  Elements=4  ZerOneIdxMode=One-based  errmode=Generate Error  FillMode=on  FillValues=0
  Variable Selector5 : dspindex/Variable Selector  NumInputs=2  rowsOrCols=Columns  IdxMode=Fixed  Elements=5  ZerOneIdxMode=One-based  errmode=Generate Error  FillMode=on  FillValues=0
  Variable Selector6 : dspindex/Variable Selector  NumInputs=2  rowsOrCols=Columns  IdxMode=Fixed  Elements=6  ZerOneIdxMode=One-based  errmode=Generate Error  FillMode=on  FillValues=0
  Variable Selector7 : dspindex/Variable Selector  NumInputs=1  rowsOrCols=Columns  IdxMode=Variable  Elements=1  ZerOneIdxMode=One-based  errmode=Generate Error  FillMode=on  FillValues=0
  eps_i : Outport
  wires:
  Variable Selector/1 -> Variable Selector3/1, Variable Selector4/1, Variable Selector6/1, Variable Selector5/1, Variable Selector2/1, Variable Selector1/1  "a(i)"
  x/1 -> Variable Selector7/1, Variable Selector2/2, Variable Selector3/2, Variable Selector4/2, Variable Selector6/2, Variable Selector5/2, Variable Selector1/2  "x"
  Constant/1 -> Variable Selector/1
  i/1 -> Variable Selector7/2, Variable Selector/3
  Variable Selector1/1 -> Divide/1  "a(i,j)"
  Variable Selector1/2 -> Subtract/1  "x(j)"
  Subtract/1 -> Divide/2
  Variable Selector2/2 -> Subtract1/1  "x(j)"
  Variable Selector2/1 -> Divide1/1  "a(i,j)"
  Subtract1/1 -> Divide1/2
  Variable Selector3/1 -> Divide2/1  "a(i,j)"
  Variable Selector3/2 -> Subtract2/1  "x(j)"
  Subtract2/1 -> Divide2/2
  Variable Selector4/1 -> Divide3/1  "a(i,j)"
  Variable Selector4/2 -> Subtract3/1  "x(j)"
  Subtract3/1 -> Divide3/2
  Variable Selector5/2 -> Subtract4/1  "x(j)"
  Subtract4/1 -> Divide4/2
  Variable Selector5/1 -> Divide4/1
  Variable Selector6/1 -> Divide5/1  "a(i,j)"
  Variable Selector7/1 -> Subtract6/2, Subtract5/2, Subtract4/2, Subtract3/2, Subtract2/2, Subtract1/2, Subtract/2  "x(i)"
  Variable Selector6/2 -> Subtract5/1  "x(j)"
  Subtract5/1 -> Divide5/2
  Divide2/1 -> Sum of Elements/3
  Divide1/1 -> Sum of Elements/2
  Divide5/1 -> Sum of Elements/6
  Divide4/1 -> Sum of Elements/5
  Divide3/1 -> Sum of Elements/4
  Divide/1 -> Sum of Elements/1
  Variable Selector/2 -> Divide6/1  "g(i)"
  Subtract6/1 -> Divide6/2
  x0/1 -> Subtract6/1
  Divide6/1 -> Sum/2
  Sum of Elements/1 -> Sum/1
  Sum/1 -> eps_i/1
  Constant1/1 -> Variable Selector/2

== system sbvf_model_2019b_local/Ideal generator /Subsystem14 ==
  u : Inport
  "y " : Inport  Port=2
  Add1 : Sum  Inputs=+++
  Gain : Gain  Gain=c*L_leader  Multiplication=Matrix(K*u)
  Gain1 : Gain  Gain=B  Multiplication=Matrix(K*u)
  Gain2 : Gain  Gain=A0  Multiplication=Matrix(K*u)
  Gain3 : Gain  Gain=C  Multiplication=Matrix(K*u)
  Integrator : Integrator  InitialCondition=x0_leader
  Subtract : Sum  Inputs=-+
  x_hat : Outport
  wires:
  Gain2/1 -> Add1/3
  Gain/1 -> Add1/2
  Integrator/1 -> x_hat/1, Gain3/1, Gain2/1  "x_hat"
  Add1/1 -> Integrator/1  "x_hat_dot"
  u/1 -> Gain1/1
  Gain1/1 -> Add1/1
  "y "/1 -> Subtract/2
  Subtract/1 -> Gain/1
  Gain3/1 -> Subtract/1
